simulink library "libMdl_InsBiasEstimator"  (R2019b)
settings: Solver=VariableStepAuto  StartTime=0.0  StopTime=10.0  RelTol=1e-3
undefined symbols (not defined in the file): mv_gyro_bias_gain
settings Model: Creator=Hanno  LastModifiedBy=Hanno

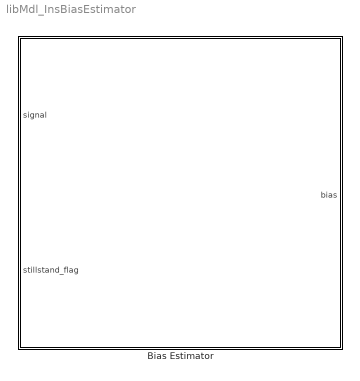
== system libMdl_InsBiasEstimator ==
  Bias Estimator : Subsystem  mask(INS Bias Estimator){mv_bias_gain=mv_gyro_bias_gain}
      mask prompts: mv_bias_gain "Bias Gain:"
      mask Display:
      | str1 = sprintf('\\color{black}{\\bfINS Bias Estimator}\n\n');
      | str2 = sprintf('Bias Gain: %0.6f\n\n',mv_bias_gain);
      | 
      | str = [str1,str2];
      | 
      | text( 0.5,0.5, ...
      |       str, ...
      |       'horizontalAlignment', 'center', ...
      |       'texmode','on' ...
      |     )

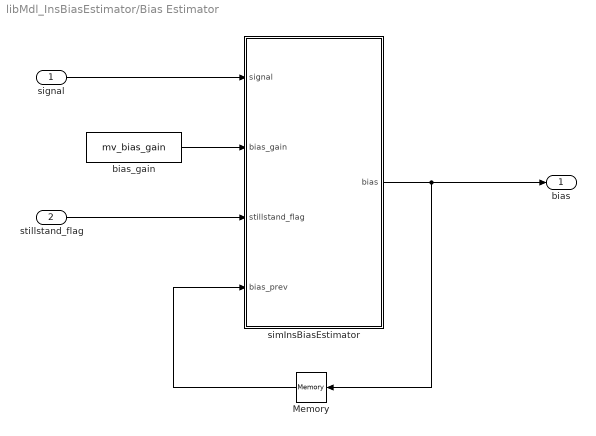
== system libMdl_InsBiasEstimator/Bias Estimator ==
  signal : Inport
  stillstand_flag : Inport  Port=2
  Memory : Memory  InheritSampleTime=on
  bias_gain : Constant  Value=mv_bias_gain
  simInsBiasEstimator : MATLAB Function  TreatAsAtomicUnit=on
  bias : Outport
  wires:
  simInsBiasEstimator/1(bias) -> Memory/1, bias/1
  Memory/1 -> simInsBiasEstimator/4(bias_prev)
  signal/1 -> simInsBiasEstimator/1(signal)
  stillstand_flag/1 -> simInsBiasEstimator/3(stillstand_flag)
  bias_gain/1 -> simInsBiasEstimator/2(bias_gain)

== matlab function libMdl_InsBiasEstimator/Bias Estimator/simInsBiasEstimator ==
  data: signal input; bias output; bias_gain input; stillstand_flag input; bias_prev input
function bias = simInsBiasEstimator(signal,bias_gain,stillstand_flag,bias_prev)

if stillstand_flag
    bias = bias_prev + bias_gain .* (signal-bias_prev);
else
    bias = bias_prev;
end % if


end % function
